simulink model "task_1_scheme"  (R2024a)
settings: Solver=FixedStepAuto  StartTime=0.0  StopTime=5.0  FixedStep=1e-4  RelTol=1e-3
libraries: matrix_library x2
settings Model: Creator=alexe  LastModifiedBy=alexe

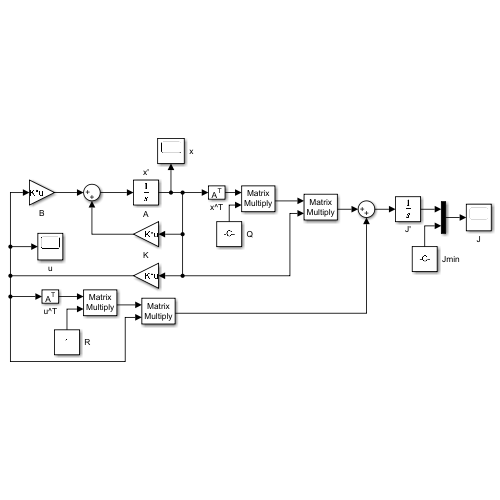
[thumbnail: Simulink's stored preview of the top-level diagram]
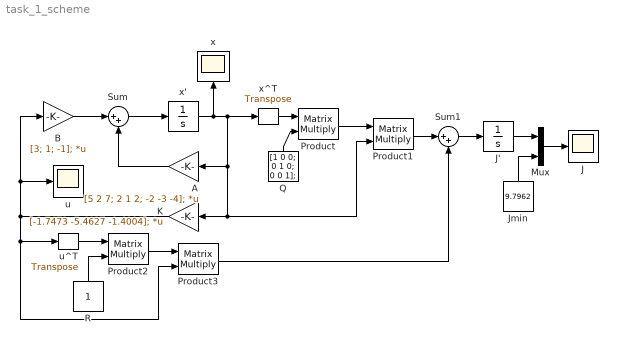
== system task_1_scheme ==
  A : Gain  Gain=[5 2 7; 2 1 2; -2 -3 -4];  Multiplication=Matrix(K*u)
  B : Gain  Gain=[3; 1; -1];  Multiplication=Matrix(K*u)
  J : Scope
  J' : Integrator
  Jmin : Constant  Value=9.7962  VectorParams1D=off
  K : Gain  Gain=[-1.7473 -5.4627 -1.4004];  Multiplication=Matrix(K*u)
  Mux : Mux  Inputs=2
  Product{,1..3} (4 alike) : Product  Multiplication=Matrix(*)
  Q : Constant  Value=[1 0 0; 0 1 0; 0 0 1];  VectorParams1D=off
  R : Constant  VectorParams1D=off
  Sum : Sum  Inputs=|++
  Sum1 : Sum  Inputs=|++
  u : Scope
  u^T : matrix_library/Transpose
  x : Scope
  x' : Integrator  InitialCondition=[1;1;1];
  x^T : matrix_library/Transpose
  wires:
  A/1 -> Sum/2
  Sum/1 -> x'/1
  B/1 -> Sum/1
  x'/1 -> x^T/1, K/1, Product1/2, A/1, x/1
  K/1 -> Product3/2, u^T/1, u/1, B/1
  x^T/1 -> Product/1
  Q/1 -> Product/2
  Product/1 -> Product1/1
  Product1/1 -> Sum1/1
  Sum1/1 -> J'/1
  u^T/1 -> Product2/1
  R/1 -> Product2/2
  Product2/1 -> Product3/1
  Product3/1 -> Sum1/2
  J'/1 -> Mux/1
  Mux/1 -> J/1
  Jmin/1 -> Mux/2
